simulink model "ASMC_2DOF_ARM"  (R2021a)
settings: Solver=VariableStepAuto  StartTime=0.0  StopTime=1  RelTol=1e-3
settings Model: Creator=Zicx  LastModifiedBy=Zicx

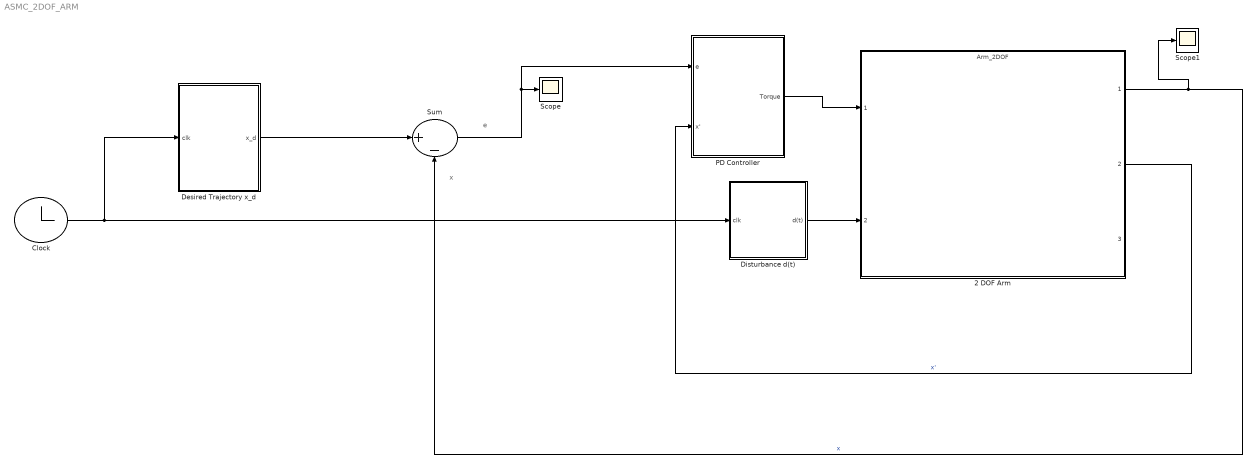
== system ASMC_2DOF_ARM ==
  note: x
  note: e
  2 DOF Arm : ModelReference  ModelNameDialog=Arm_2DOF  SimulationMode=Normal  ModelReferenceVersion=1.23
  Clock : Clock
  Desired Trajectory x_d : Subsystem
  Disturbance d(t) : Subsystem
  PD Controller : Subsystem
  Scope : Scope
  Scope1 : Scope
  Sum : Sum  Inputs=|+-
  wires:
  Clock/1 -> Disturbance d(t)/1(clk), Desired Trajectory x_d/1(clk)
  Desired Trajectory x_d/1(x_d) -> Sum/1
  2 DOF Arm/1 -> Scope1/1, Sum/2  "x"
  Sum/1 -> Scope/1, PD Controller/1(e)
  Disturbance d(t)/1(d(t)) -> 2 DOF Arm/2
  PD Controller/1(Torque) -> 2 DOF Arm/1
  2 DOF Arm/2 -> PD Controller/2(x')  "x'"

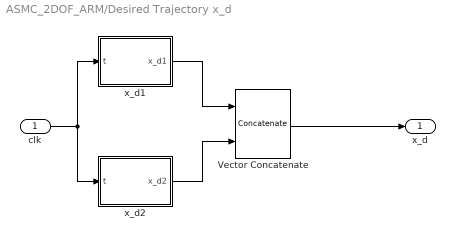
== system ASMC_2DOF_ARM/Desired Trajectory x_d ==
  clk : Inport
  Vector Concatenate : Concatenate
  x_d1 : MATLAB Function  TreatAsAtomicUnit=on
  x_d2 : MATLAB Function  TreatAsAtomicUnit=on
  x_d : Outport
  wires:
  clk/1 -> x_d2/1(t), x_d1/1(t)
  x_d1/1(x_d1) -> Vector Concatenate/1
  Vector Concatenate/1 -> x_d/1
  x_d2/1(x_d2) -> Vector Concatenate/2

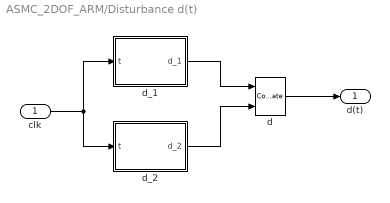
== system ASMC_2DOF_ARM/Disturbance d(t) ==
  clk : Inport
  d : Concatenate
  d_1 : MATLAB Function  TreatAsAtomicUnit=on
  d_2 : MATLAB Function  TreatAsAtomicUnit=on
  d(t) : Outport
  wires:
  d/1 -> d(t)/1
  clk/1 -> d_2/1(t), d_1/1(t)
  d_1/1(d_1) -> d/1
  d_2/1(d_2) -> d/2

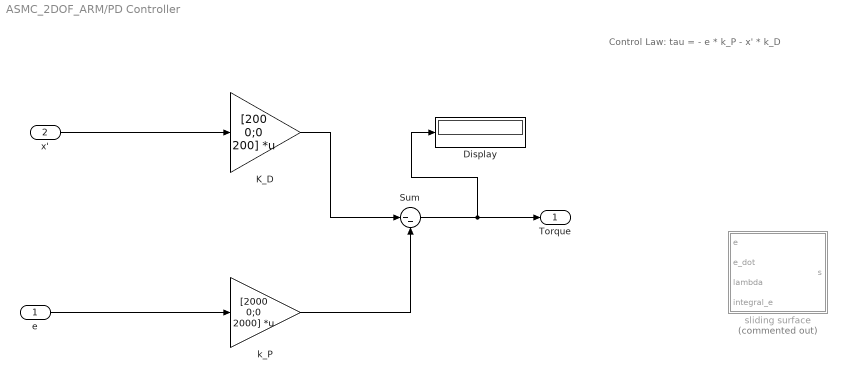
== system ASMC_2DOF_ARM/PD Controller ==
  note: Control Law:
      |
      | tau = - e * k_P - x' * k_D
  e : Inport
  x' : Inport  Port=2
  Display : Display
  K_D : Gain  Gain=[200 0;0 200]  Multiplication=Matrix(K*u) (u vector)
  Sum : Sum  Inputs=|--
  k_P : Gain  Gain=[2000 0;0 2000]  Multiplication=Matrix(K*u) (u vector)
  sliding surface : MATLAB Function  Commented=on  TreatAsAtomicUnit=on
  Torque : Outport
  wires:
  e/1 -> k_P/1
  K_D/1 -> Sum/1
  k_P/1 -> Sum/2
  Sum/1 -> Display/1, Torque/1
  x'/1 -> K_D/1

== matlab function ASMC_2DOF_ARM/Desired Trajectory x_d/x_d2 ==
  data: t input; x_d2 output
function x_d2 = fcn(t)

x_d2 = pi/6 * (1 - cos(2 * pi * t) + sin(1.5 * pi * t));

== matlab function ASMC_2DOF_ARM/Desired Trajectory x_d/x_d1 ==
  data: t input; x_d1 output
function x_d1 = fcn(t)

x_d1 = pi/6 * (1 - cos(1.5 * pi * t) + sin(pi * t));

== matlab function ASMC_2DOF_ARM/PD Controller/sliding surface ==
  data: e input; s output; e_dot input; lambda input; integral_e input
function s = fcn(e, e_dot, lambda, integral_e)

s = e_dot + 2 * lambda * e + (lambda^2) * integral_e;

== matlab function ASMC_2DOF_ARM/Disturbance d(t)/d_1 ==
  data: t input; d_1 output
function d_1 = fcn(t)

d_1 = 300* cos(1.7*pi*(t+12)) + 270* sin(pi*t);

== matlab function ASMC_2DOF_ARM/Disturbance d(t)/d_2 ==
  data: t input; d_2 output
function d_2 = fcn(t)

d_2 = 250 * sin(1.35*pi*(t + 12)) + 300 * cos(2*t);
